simulink model "dynamical_system_question_2"  (R2023b)
settings: Solver=VariableStepAuto  StartTime=0.0  StopTime=50  RelTol=1e-3
settings Model: Creator=orife  LastModifiedBy=orife

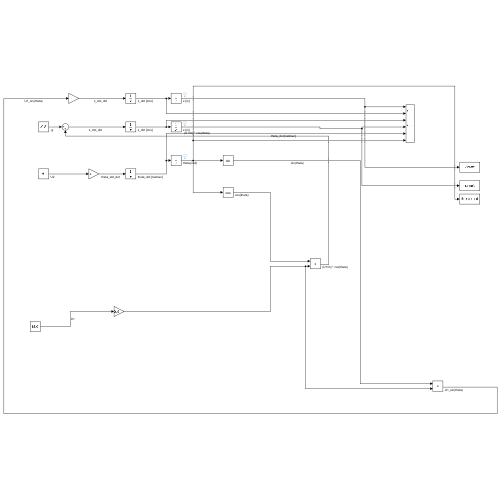
[thumbnail: Simulink's stored preview of the top-level diagram]
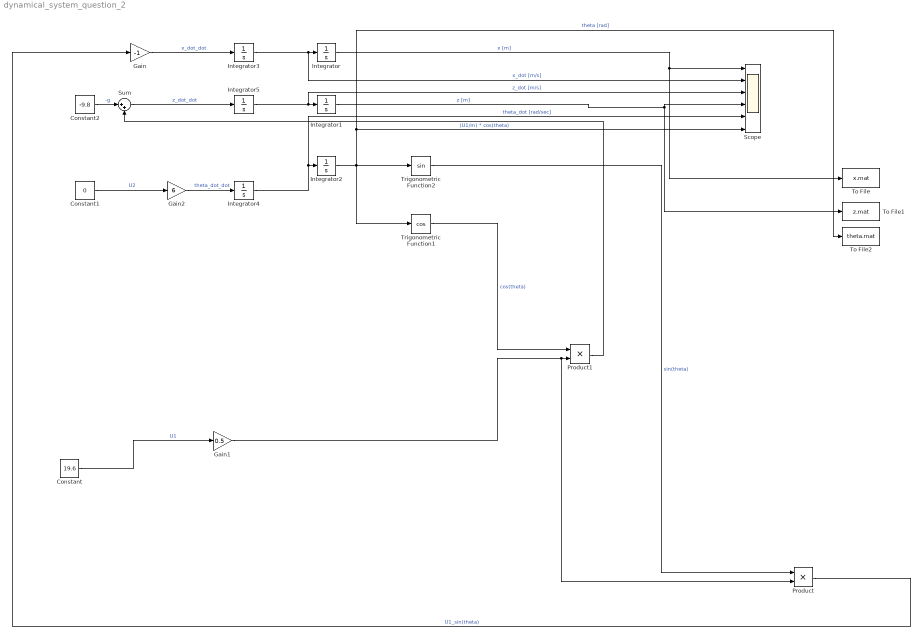
== system dynamical_system_question_2 ==
  Constant : Constant  Value=19.6
  Constant1 : Constant  Value=0
  Constant2 : Constant  Value=-9.8
  Gain : Gain  Gain=-1
  Gain1 : Gain  Gain=0.5
  Gain2 : Gain  Gain=6
  Integrator{,1,3..5} (5 alike) : Integrator
  Integrator2 : Integrator  InitialCondition=(4/180)*pi
  Product : Product
  Product1 : Product
  Scope : Scope  NumInputPorts=6
  Sum : Sum  Inputs=|++
  To File : ToFile  Filename=x.mat  SaveFormat=Timeseries
  To File1 : ToFile  Filename=z.mat  SaveFormat=Timeseries
  To File2 : ToFile  Filename=theta.mat  SaveFormat=Timeseries
  Trigonometric Function1 : Trigonometry  Operator=cos
  Trigonometric Function2 : Trigonometry
  wires:
  Integrator2/1 -> To File2/1, Scope/6, Trigonometric Function1/1, Trigonometric Function2/1  "theta [rad]"
  Integrator3/1 -> Scope/2, Integrator/1  "x_dot [m/s]"
  Trigonometric Function2/1 -> Product/1  "sin(theta)"
  Constant/1 -> Gain1/1  "U1"
  Product/1 -> Gain/1  "U1_sin(theta)"
  Gain/1 -> Integrator3/1  "x_dot_dot"
  Integrator4/1 -> Integrator2/1, Scope/5  "theta_dot [rad/sec]"
  Integrator5/1 -> Scope/3, Integrator1/1  "z_dot [m/s]"
  Sum/1 -> Integrator5/1  "z_dot_dot"
  Product1/1 -> Sum/2  "(U1/m) * cos(theta)"
  Constant2/1 -> Sum/1  "-g"
  Constant1/1 -> Gain2/1  "U2"
  Gain2/1 -> Integrator4/1  "theta_dot_dot"
  Integrator1/1 -> To File1/1, Scope/4  "z [m]"
  Integrator/1 -> To File/1, Scope/1  "x [m]"
  Trigonometric Function1/1 -> Product1/1  "cos(theta)"
  Gain1/1 -> Product/2, Product1/2
